simulink model "W3Q3"  (R2020b)
settings: Solver=ode45  StartTime=0.0  StopTime=100  RelTol=1e-3
values from neighbouring files (symbols this model uses):
  b1 = 330    [var_values.m]
  b2 = 14000    [var_values.m]
  k1 = 50000.0    [parameter.sldd]    (also in var_values.m = 75000)
  k2 = 500000.0    [parameter.sldd]    (also in var_values.m = 480000)
  m1 = 2500.0    [parameter.sldd]    (also in var_values.m = 2800)
  m2 = 250.0    [parameter.sldd]    (also in var_values.m = 370)
settings Model: DataDictionary=parameter.sldd  Creator=VIVEK  LastModifiedBy=VIVEK

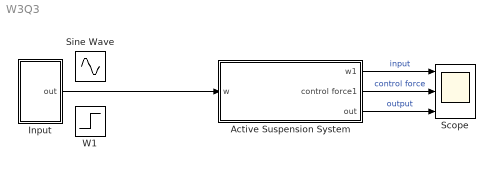
== system W3Q3 ==
  Active Suspension System : Subsystem
  Input : Subsystem
  Scope : Scope  NumInputPorts=3
  Sine Wave : Sin  SampleTime=0
  W1 : Step  Time=0  After=0
  wires:
  Active Suspension System/2(control force1) -> Scope/2  "control force"
  Active Suspension System/1(w1) -> Scope/1  "input"
  Active Suspension System/3(out) -> Scope/3  "output"
  Input/1(out) -> Active Suspension System/1(w)

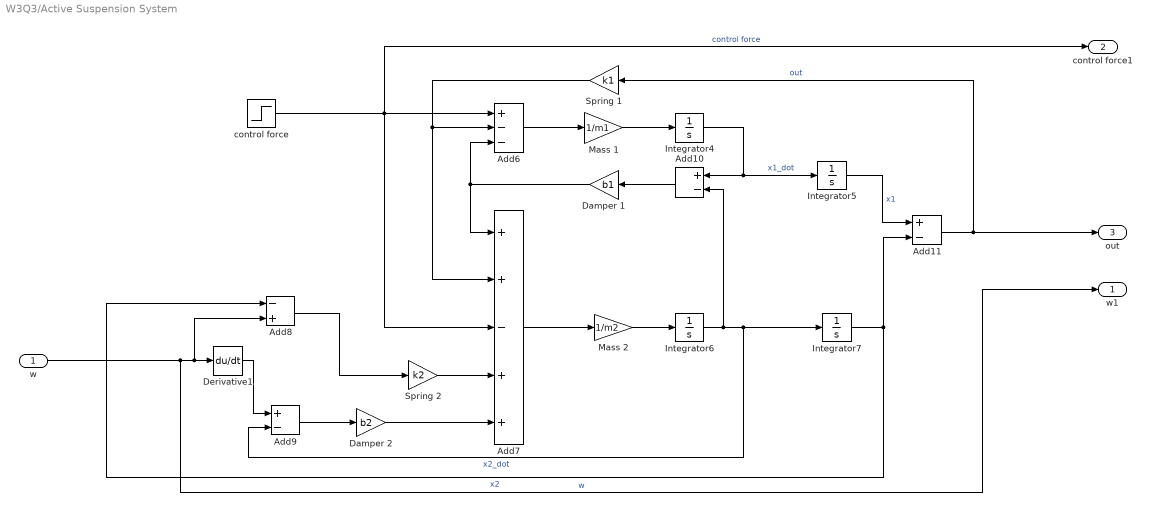
== system W3Q3/Active Suspension System ==
  w : Inport
  Add10 : Sum  Inputs=+-
  Add11 : Sum  Inputs=+-
  Add6 : Sum  Inputs=+--
  Add7 : Sum  Inputs=++-++
  Add8 : Sum  Inputs=-+
  Add9 : Sum  Inputs=+-
  Damper 1 : Gain  Gain=b1
  Damper 2 : Gain  Gain=b2
  Derivative1 : Derivative
  Integrator{4..7} (4 alike) : Integrator
  Mass 1 : Gain  Gain=1/m1
  Mass 2 : Gain  Gain=1/m2
  Spring 1 : Gain  Gain=k1
  Spring 2 : Gain  Gain=k2
  control force : Step  SampleTime=0
  w1 : Outport
  control force1 : Outport  Port=2
  out : Outport  Port=3
  wires:
  Integrator6/1 -> Integrator7/1, Add9/2, Add10/2  "x2_dot"
  control force/1 -> Add7/3, control force1/1, Add6/1  "control force"
  Spring 2/1 -> Add7/4
  Damper 2/1 -> Add7/5
  Add11/1 -> out/1, Spring 1/1  "out"
  w/1 -> w1/1, Derivative1/1, Add8/2  "w"
  Damper 1/1 -> Add7/1, Add6/3
  Add8/1 -> Spring 2/1
  Integrator7/1 -> Add11/2, Add8/1  "x2"
  Spring 1/1 -> Add7/2, Add6/2
  Add9/1 -> Damper 2/1
  Add7/1 -> Mass 2/1
  Integrator5/1 -> Add11/1  "x1"
  Add6/1 -> Mass 1/1
  Mass 1/1 -> Integrator4/1
  Mass 2/1 -> Integrator6/1
  Integrator4/1 -> Integrator5/1, Add10/1  "x1_dot"
  Derivative1/1 -> Add9/1
  Add10/1 -> Damper 1/1

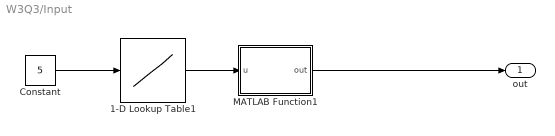
== system W3Q3/Input ==
  1-D Lookup Table1 : Lookup_n-D  NumberOfTableDimensions=1  BreakpointsForDimension1=[0:10]  Table=[1,1.1,1.2,1.3,1.4,1.5,1.6,1.7,1.8,1.9,2]  InternalRulePriority=Speed  RndMeth=Simplest  InputSameDT=on
  Constant : Constant  Value=5
  MATLAB Function1 : MATLAB Function  TreatAsAtomicUnit=on
  out : Outport
  wires:
  Constant/1 -> 1-D Lookup Table1/1
  1-D Lookup Table1/1 -> MATLAB Function1/1(u)
  MATLAB Function1/1(out) -> out/1

== matlab function W3Q3/Input/MATLAB Function1 ==
  data: u input; out output
function out = fcn(u)
if(u>1.5)
    out=1;
else
    out=u;

end
